simulink model "untitled"  (R2023a)
settings: Solver=VariableStepAuto  StartTime=0.0  StopTime=10.0  RelTol=1e-3
values from neighbouring files (symbols this model uses):
  K = 4.7    [matlab.mat]    (also in zad1.m; zad10.m = inv(M' * Gamma * M + Alpha) * M' * Gamma; zad10b.m = inv(M' * Gamma * M + Alpha) * M' * Gamma; zad4.m = inv(M' * Gamma * M + Alpha) * M' * Gamma)
  T1 = 1.78    [matlab.mat]    (also in zad1.m; zad10.m; zad10b.m; zad6dmc.m)
  T2 = 5.13    [matlab.mat]    (also in zad1.m; zad10.m; zad10b.m; zad6dmc.m)
  Td = 0    [matlab.mat]    (also in zad2.m; zad2dyskr.m = 1.94; zad3.m = 1.94; zad3popraw.m)
  Ti = inf    [matlab.mat]    (also in zad2.m; zad2dyskr.m = 7.95; zad3.m = 7.95; zad6pid.m = 7.95)
undefined symbols (not defined in the file or in its folder): Kpd
settings Model: Creator=pkutyl  LastModifiedBy=pkutyl

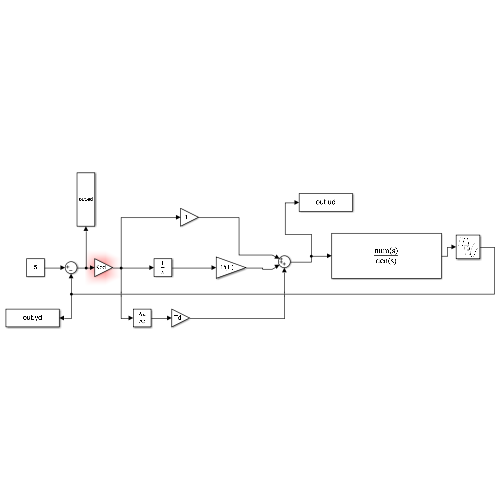
[thumbnail: Simulink's stored preview of the top-level diagram]
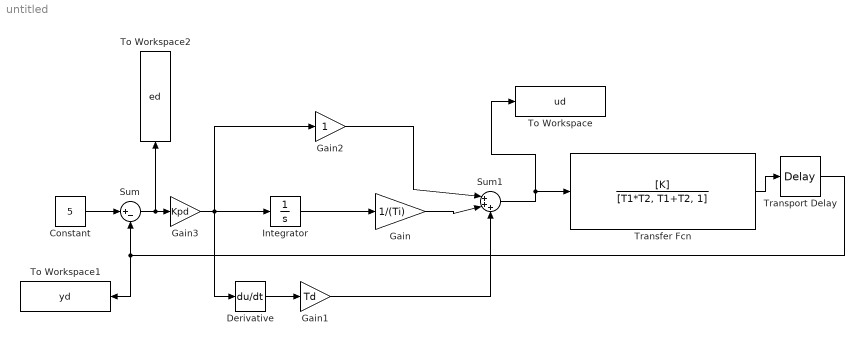
== system untitled ==
  Constant : Constant  Value=5
  Derivative : Derivative
  Gain : Gain  Gain=1/(Ti)
  Gain1 : Gain  Gain=Td
  Gain2 : Gain
  Gain3 : Gain  Gain=Kpd
  Integrator : Integrator
  Sum : Sum  Inputs=|+-
  Sum1 : Sum  Inputs=|+++
  To Workspace : ToWorkspace  VariableName=ud  SaveFormat=Structure With Time  SampleTime=-1
  To Workspace1 : ToWorkspace  VariableName=yd  SaveFormat=Structure With Time  SampleTime=-1
  To Workspace2 : ToWorkspace  VariableName=ed  SaveFormat=Structure With Time  SampleTime=-1
  Transfer Fcn : TransferFcn  Numerator=[K]  Denominator=[T1*T2, T1+T2, 1]
  Transport Delay : TransportDelay  DelayTime=5
  wires:
  Integrator/1 -> Gain/1
  Gain1/1 -> Sum1/3
  Transport Delay/1 -> To Workspace1/1, Sum/2
  Sum/1 -> To Workspace2/1, Gain3/1
  Gain3/1 -> Integrator/1, Gain2/1, Derivative/1
  Transfer Fcn/1 -> Transport Delay/1
  Constant/1 -> Sum/1
  Gain/1 -> Sum1/2
  Sum1/1 -> To Workspace/1, Transfer Fcn/1
  Derivative/1 -> Gain1/1
  Gain2/1 -> Sum1/1
